simulink model "bh_proto_balance"  (R2017a)
settings: Solver=ode45  StartTime=0.0  StopTime=2  FixedStep=0.001  RelTol=1e-5  EnableMultiTasking=on
values from neighbouring files (symbols this model uses):
  L3y = res_T.L3y    [bh_pend_solve_ODE_sys.m]    (also in bh_pend_solve_ODE_sys_custom.m)
  m = res_T.mass3    [bh_pend_solve_ODE_sys_custom.m]
  N = 1 + N_steps    [bh_pend_solve_ODE_sys_custom.m]
undefined symbols (not defined in the file or in its folder): L3x, L3z, X, Y, Z
libraries: sm_lib x13, nesl_utility x8, simulink_extras x5
settings Model: Creator=bhorton  LastModifiedBy=bhorton
settings SolverCC: ZeroCrossAlgorithm=Adaptive
settings OptimizationCC: LifeSpan=inf
settings DebuggingCC: SFUnexpectedBacktrackingDiag=warning  SFNoUnconditionalDefaultTransitionDiag=warning  SFExecutionAtInitializationDiag=none
settings GRTTargetCC: TargetLangStandard=C89/C90 (ANSI)
settings ConfigComp: CovMetricSettings=dw  CovHtmlReporting=on  CovSaveCumulativeToWorkspaceVar=on  CovSaveSingleToWorkspaceVar=on  CovExternalEMLEnable=off
settings SimscapeCC: SimscapeLogDataHistory=10000  SelectedTab=Simscape Multibody
settings ExplorerConfigSet: InternalSimMechanicsExplorerSettings="<ExplorerConfiguration><canonicalview>default</canonicalview><AnimationSetting><BasePlaybackSpeed>1.0</BasePlaybackSpeed><PlaybackSpeedFactor>1.0</PlaybackSpeedFactor></AnimationSetting><TilePanel><TileInfo><Tiles Columns=\"1\" Count=\"1\" Rows=\"1\"><Column Left=\"2\" Weight=\"1\"/><Column Left=\"1585\" Weight=\"0.5\"/><Row Top=\"2\" Weight=\"1\"/><Row Top=\"911\" Weight=\"0.5005\"/><Tile Height=\"1\" Width=\"1\" X=\"0\" Y=\"0\"/></Tiles></TileInfo><SceneInfo><SceneViewer><BGColor><R>0.60000002384185791</R><G>0.60000002384185791</G><B>0.60000002384185791</B></BGColor><Camera><DoPerspective>off</DoPerspective><Position><X>0.97226610796774449</X><Y>0.24871023220719646</Y><Z>0.19848014681163439</Z></Position><Center><X>-1.1885447515069814e-08</X><Y>0.12499999495795672</Y><Z>-1.7810067587387124e-09</Z></Center><Up><X>-0.2183009159559649</X><Y>0.17550270816811642</Y><Z>0.9599705774233106</Z></Up><ViewLimDist>1</ViewLimDist><YLim>0.073618170266836078</YLim><XLim>0.12874999999999998</XLim></Camera></SceneViewer></SceneInfo></TilePanel><MechEditorPanel><Cameras/><GfxPanelCameraMap/><VideoCreator><PlaybackSpeedRatio>1.0</PlaybackSpeedRatio><FrameRate>30</FrameRate><VideoFormat>Motion JPEG AVI</VideoFormat><FrameSize>auto</FrameSize></VideoCreator></MechEditorPanel></ExplorerConfiguration>"

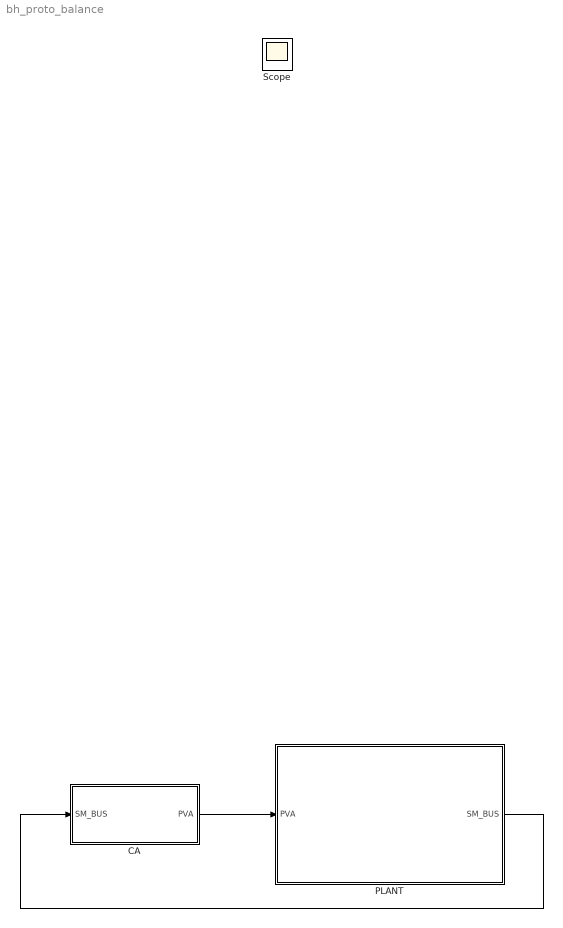
== system bh_proto_balance ==
  CA : Subsystem
  PLANT : Subsystem
  Scope : Scope
  wires:
  PLANT/1(SM_BUS) -> CA/1(SM_BUS)
  CA/1(PVA) -> PLANT/1(PVA)

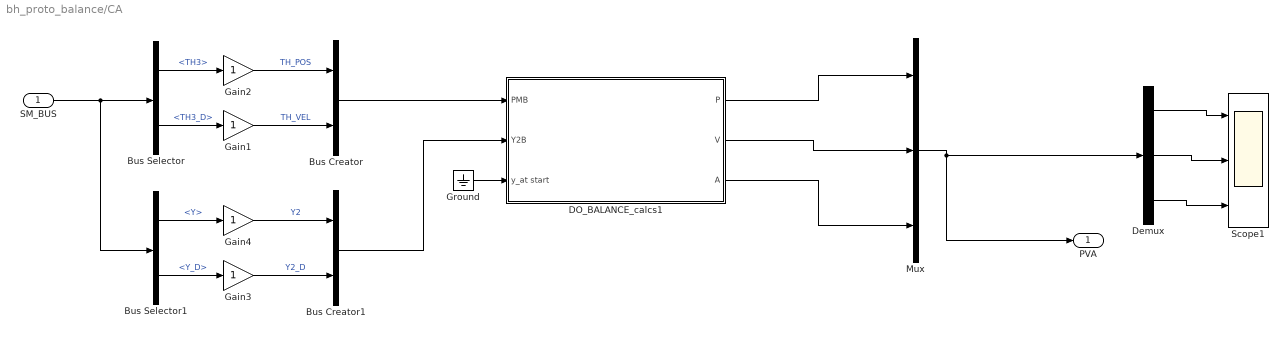
== system bh_proto_balance/CA ==
  SM_BUS : Inport
  Bus Creator : BusCreator  Inputs=2
  Bus Creator1 : BusCreator  Inputs=2
  Bus Selector : BusSelector  OutputSignals=TH3,TH3_D
  Bus Selector1 : BusSelector  OutputSignals=Y,Y_D
  DO_BALANCE_calcs1 : Subsystem  TreatAsAtomicUnit=on
  Demux : Demux  Outputs=3
  Gain{1..4} (4 alike) : Gain
  Ground : Ground
  Mux : Mux  Inputs=3
  Scope1 : Scope  NumInputPorts=3
  PVA : Outport
  wires:
  Mux/1 -> Demux/1, PVA/1
  Demux/3 -> Scope1/3
  Demux/2 -> Scope1/2
  Demux/1 -> Scope1/1
  Bus Selector/1 -> Gain2/1  "<TH3>"
  Bus Selector/2 -> Gain1/1  "<TH3_D>"
  Gain1/1 -> Bus Creator/2  "TH_VEL"
  Gain2/1 -> Bus Creator/1  "TH_POS"
  Bus Selector1/1 -> Gain4/1  "<Y>"
  Gain4/1 -> Bus Creator1/1  "Y2"
  Gain3/1 -> Bus Creator1/2  "Y2_D"
  Bus Selector1/2 -> Gain3/1  "<Y_D>"
  SM_BUS/1 -> Bus Selector1/1, Bus Selector/1
  Bus Creator/1 -> DO_BALANCE_calcs1/1(PMB)
  Bus Creator1/1 -> DO_BALANCE_calcs1/2(Y2B)
  DO_BALANCE_calcs1/1(P) -> Mux/1
  Ground/1 -> DO_BALANCE_calcs1/3(y_at start)
  DO_BALANCE_calcs1/2(V) -> Mux/2
  DO_BALANCE_calcs1/3(A) -> Mux/3

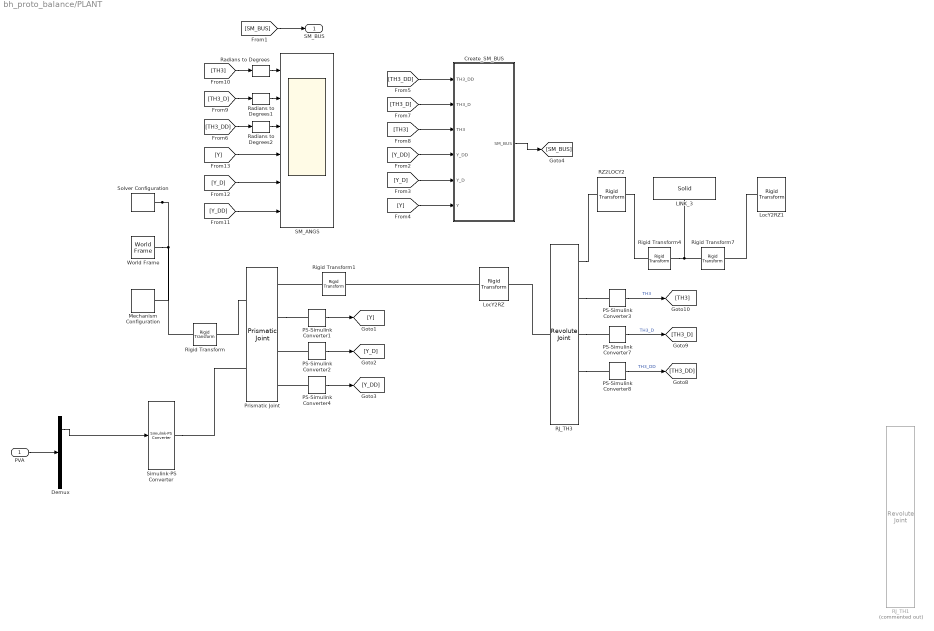
== system bh_proto_balance/PLANT ==
  PVA : Inport
  Create_SM_BUS : Subsystem
  Demux : Demux  Outputs=3
  LINK_3 : sm_lib/Body Elements/Solid  InertiaType=CalculateFromGeometry  Mass=1  MassUnits=kg  CenterOfMass=[0 0 0]  CenterOfMassUnits=m  MomentsOfInertia=[1 1 1]  MomentsOfInertiaUnits=kg*m^2  ProductsOfInertia=[0 0 0]  ProductsOfInertiaUnits=kg*m^2  DensityBased=on  Density=density  DensityUnits=kg/(m^3)  DoExposeReferenceFrame=on  SerializedFrames=<Frames/>  GraphicType=FromGeometry  MarkerShape=Sphere  MarkerSize=10  GraphicVisPropType=SimpleVisualProperties  GraphicDiffuseColor=[1.0 0.8 0.4]  GraphicSpecularColor=[0.5 0.5 0.5 1.0]  GraphicAmbientColor=[0.15 0.15 0.15 1.0]  GraphicEmissiveColor=[0.0 0.0 0.0 1.0]  GraphicShininess=75  GraphicOpacity=1.0  GeometryShape=Brick  RectangleSize=[1 1]  RectangleSizeUnits=m  BrickDimensions=[L3x, L3y, L3z ]  BrickDimensionUnits=m  CylinderRadius=1  CylinderRadiusUnits=m  CylinderLength=1  CylinderLengthUnits=m  SphereRadius=1  SphereRadiusUnits=m  EllipsoidRadii=[1 1 1]  EllipsoidRadiiUnits=m  ExtrusionCrossSection=[1 1; -1 1; -1 -1; 1 -1]  ExtrusionCrossSectionUnits=m  ExtrusionLength=1  ExtrusionLengthUnits=m  PolygonNumSides=3  PolygonOuterRadius=1  PolygonOuterRadiusUnits=m  ExtGeomFileType=STEP  ExtGeomFileUnits=m  RevolutionCrossSection=[1 1; 1 -1; 2 -1; 2 1]  RevolutionCrossSectionUnits=m  RevolutionExtent=Full  RevolutionAngle=180  RevolutionAngleUnits=deg
  LocY2RZ : sm_lib/Frames and Transforms/Rigid Transform  TranslationMethod=None  TranslationStandardOffset=0  TranslationLengthUnit=m  TranslationStandardAxis=+Z  TranslationCartesianOffset=[0 0 0]  TranslationROffset=0  TranslationROffsetUnits=m  TranslationZOffset=0  TranslationZOffsetUnits=m  TranslationThetaOffset=0  TranslationThetaOffsetUnits=deg  RotationMethod=AlignedAxes  RotationAngleUnits=deg  RotationStandardAxis=+Z  RotationAngle=0.0  RotationArbitraryAxis=[0 0 1]  FollAlignAxisA=+X  BaseAlignAxisA=+Y  FollAlignAxisB=+Y  BaseAlignAxisB=+Z  RotationSequenceAxes=FollowerAxes  RotationSequence=XYX  RotationSequenceAngles=[0 0 0]  RotationSequenceAnglesUnits=deg  RotationMatrix=[1 0 0; 0 1 0; 0 0 1]
  LocY2RZ1 : sm_lib/Frames and Transforms/Rigid Transform  TranslationMethod=None  TranslationStandardOffset=0  TranslationLengthUnit=m  TranslationStandardAxis=+Z  TranslationCartesianOffset=[0 0 0]  TranslationROffset=0  TranslationROffsetUnits=m  TranslationZOffset=0  TranslationZOffsetUnits=m  TranslationThetaOffset=0  TranslationThetaOffsetUnits=deg  RotationMethod=AlignedAxes  RotationAngleUnits=deg  RotationStandardAxis=+Z  RotationAngle=0.0  RotationArbitraryAxis=[0 0 1]  FollAlignAxisA=+X  BaseAlignAxisA=+Y  FollAlignAxisB=+Y  BaseAlignAxisB=+Z  RotationSequenceAxes=FollowerAxes  RotationSequence=XYX  RotationSequenceAngles=[0 0 0]  RotationSequenceAnglesUnits=deg  RotationMatrix=[1 0 0; 0 1 0; 0 0 1]
  Mechanism Configuration : sm_lib/Utilities/Mechanism Configuration  UniformGravity=Constant  GravityVector=[0 0 -9.80665 ]  GravityUnits=m/s^2  LinearizationDelta=1e-4
  PS-Simulink Converter1 : nesl_utility/PS-Simulink Converter  PhysicalDomain=network_engine_domain  SubClassName=ps_output  LeftPortType=input  RightPortType=output  PseudoPeriodic=off  Frequencies=[]  Unit=m  AffineConversion=off
  PS-Simulink Converter2 : nesl_utility/PS-Simulink Converter  PhysicalDomain=network_engine_domain  SubClassName=ps_output  LeftPortType=input  RightPortType=output  PseudoPeriodic=off  Frequencies=[]  Unit=m/s  AffineConversion=off
  PS-Simulink Converter3 : nesl_utility/PS-Simulink Converter  PhysicalDomain=network_engine_domain  SubClassName=ps_output  LeftPortType=input  RightPortType=output  PseudoPeriodic=off  Frequencies=[]  Unit=rad  AffineConversion=off
  PS-Simulink Converter4 : nesl_utility/PS-Simulink Converter  PhysicalDomain=network_engine_domain  SubClassName=ps_output  LeftPortType=input  RightPortType=output  PseudoPeriodic=off  Frequencies=[]  Unit=m/s^2  AffineConversion=off
  PS-Simulink Converter7 : nesl_utility/PS-Simulink Converter  PhysicalDomain=network_engine_domain  SubClassName=ps_output  LeftPortType=input  RightPortType=output  PseudoPeriodic=off  Frequencies=[]  Unit=rad/s  AffineConversion=off
  PS-Simulink Converter8 : nesl_utility/PS-Simulink Converter  PhysicalDomain=network_engine_domain  SubClassName=ps_output  LeftPortType=input  RightPortType=output  PseudoPeriodic=off  Frequencies=[]  Unit=rad/s^2  AffineConversion=off
  Prismatic Joint : sm_lib/Joints/Prismatic Joint  SenseConstraintForce=off  SenseConstraintForceX=off  SenseConstraintForceY=off  SenseConstraintForceZ=off  SenseConstraintTorque=off  SenseConstraintTorqueX=off  SenseConstraintTorqueY=off  SenseConstraintTorqueZ=off  SenseTotalForce=off  SenseTotalForceX=off  SenseTotalForceY=off  SenseTotalForceZ=off  SenseTotalTorque=off  SenseTotalTorqueX=off  SenseTotalTorqueY=off  SenseTotalTorqueZ=off  CompositeWrenchDir=FollowerOnBase  CompositeWrenchFrame=BaseFrame  EquilibriumPosition=0  EquilibriumPositionUnits=m  SpringStiffness=0  SpringStiffnessUnits=N/m  DampingCoefficient=0  DampingCoefficientUnits=N/(m/s)  TorqueActuationMode=ComputedTorque  MotionActuationMode=InputMotion  SensePosition=on  SenseVelocity=on  SenseAcceleration=on  SenseTorqueForce=off  PositionTargetSpecify=on  PositionTargetPriority=High  PositionTargetValue=0  PositionTargetValueUnits=m  VelocityTargetSpecify=on  VelocityTargetPriority=High  VelocityTargetValue=0  VelocityTargetValueUnits=m/s
  RJ_TH1 : sm_lib/Joints/Revolute Joint  Commented=on  SenseConstraintForce=on  SenseConstraintForceX=off  SenseConstraintForceY=off  SenseConstraintForceZ=off  SenseConstraintTorque=off  SenseConstraintTorqueX=off  SenseConstraintTorqueY=off  SenseConstraintTorqueZ=off  SenseTotalForce=off  SenseTotalForceX=off  SenseTotalForceY=off  SenseTotalForceZ=off  SenseTotalTorque=off  SenseTotalTorqueX=off  SenseTotalTorqueY=off  SenseTotalTorqueZ=off  CompositeWrenchDir=BaseOnFollower  CompositeWrenchFrame=BaseFrame  EquilibriumPosition=0  EquilibriumPositionUnits=deg  SpringStiffness=0  SpringStiffnessUnits=N*m/deg  DampingCoefficient=b3_damp  DampingCoefficientUnits=N*m/(rad/s)  TorqueActuationMode=NoTorque  MotionActuationMode=ComputedMotion  SensePosition=on  SenseVelocity=on  SenseAcceleration=on  SenseTorqueForce=off  PositionTargetSpecify=on  PositionTargetPriority=Low  PositionTargetValue=80  PositionTargetValueUnits=deg  VelocityTargetSpecify=on  VelocityTargetPriority=High  VelocityTargetValue=-100  VelocityTargetValueUnits=deg/s
      settings: AttributesFormatString=|
      | %<DampingCoefficient>
      | %<PositionTargetValue>
      | %<VelocityTargetValue>
  RJ_TH3 : sm_lib/Joints/Revolute Joint  SenseConstraintForce=on  SenseConstraintForceX=off  SenseConstraintForceY=off  SenseConstraintForceZ=off  SenseConstraintTorque=off  SenseConstraintTorqueX=off  SenseConstraintTorqueY=off  SenseConstraintTorqueZ=off  SenseTotalForce=off  SenseTotalForceX=off  SenseTotalForceY=off  SenseTotalForceZ=off  SenseTotalTorque=off  SenseTotalTorqueX=off  SenseTotalTorqueY=off  SenseTotalTorqueZ=off  CompositeWrenchDir=BaseOnFollower  CompositeWrenchFrame=BaseFrame  EquilibriumPosition=0  EquilibriumPositionUnits=deg  SpringStiffness=0  SpringStiffnessUnits=N*m/deg  DampingCoefficient=b3_damp  DampingCoefficientUnits=N*m/(rad/s)  TorqueActuationMode=NoTorque  MotionActuationMode=ComputedMotion  SensePosition=on  SenseVelocity=on  SenseAcceleration=on  SenseTorqueForce=off  PositionTargetSpecify=on  PositionTargetPriority=Low  PositionTargetValue=80  PositionTargetValueUnits=deg  VelocityTargetSpecify=on  VelocityTargetPriority=High  VelocityTargetValue=-350  VelocityTargetValueUnits=deg/s
      settings: AttributesFormatString=|
      | %<DampingCoefficient>
      | %<PositionTargetValue>
      | %<VelocityTargetValue>
  RZ2LOCY2 : sm_lib/Frames and Transforms/Rigid Transform  TranslationMethod=None  TranslationStandardOffset=0  TranslationLengthUnit=m  TranslationStandardAxis=+Z  TranslationCartesianOffset=[0 0 0]  TranslationROffset=0  TranslationROffsetUnits=m  TranslationZOffset=0  TranslationZOffsetUnits=m  TranslationThetaOffset=0  TranslationThetaOffsetUnits=deg  RotationMethod=AlignedAxes  RotationAngleUnits=deg  RotationStandardAxis=+Z  RotationAngle=0.0  RotationArbitraryAxis=[0 0 1]  FollAlignAxisA=+Y  BaseAlignAxisA=+X  FollAlignAxisB=+X  BaseAlignAxisB=+Z  RotationSequenceAxes=FollowerAxes  RotationSequence=XYX  RotationSequenceAngles=[0 0 0]  RotationSequenceAnglesUnits=deg  RotationMatrix=[1 0 0; 0 1 0; 0 0 1]
  Radians to Degrees : simulink_extras/Transformations/Radians to Degrees
  Radians to Degrees1 : simulink_extras/Transformations/Radians to Degrees
  Radians to Degrees2 : simulink_extras/Transformations/Radians to Degrees
  Rigid Transform : sm_lib/Frames and Transforms/Rigid Transform  TranslationMethod=None  TranslationStandardOffset=0  TranslationLengthUnit=m  TranslationStandardAxis=+Z  TranslationCartesianOffset=[0 0 0]  TranslationROffset=0  TranslationROffsetUnits=m  TranslationZOffset=0  TranslationZOffsetUnits=m  TranslationThetaOffset=0  TranslationThetaOffsetUnits=deg  RotationMethod=AlignedAxes  RotationAngleUnits=deg  RotationStandardAxis=+Z  RotationAngle=0.0  RotationArbitraryAxis=[0 0 1]  FollAlignAxisA=+X  BaseAlignAxisA=+X  FollAlignAxisB=+Z  BaseAlignAxisB=+Y  RotationSequenceAxes=FollowerAxes  RotationSequence=XYX  RotationSequenceAngles=[0 0 0]  RotationSequenceAnglesUnits=deg  RotationMatrix=[1 0 0; 0 1 0; 0 0 1]
  Rigid Transform1 : sm_lib/Frames and Transforms/Rigid Transform  TranslationMethod=None  TranslationStandardOffset=0  TranslationLengthUnit=m  TranslationStandardAxis=+Z  TranslationCartesianOffset=[0 0 0]  TranslationROffset=0  TranslationROffsetUnits=m  TranslationZOffset=0  TranslationZOffsetUnits=m  TranslationThetaOffset=0  TranslationThetaOffsetUnits=deg  RotationMethod=AlignedAxes  RotationAngleUnits=deg  RotationStandardAxis=+Z  RotationAngle=0.0  RotationArbitraryAxis=[0 0 1]  FollAlignAxisA=+X  BaseAlignAxisA=+X  FollAlignAxisB=+Y  BaseAlignAxisB=+Z  RotationSequenceAxes=FollowerAxes  RotationSequence=XYX  RotationSequenceAngles=[0 0 0]  RotationSequenceAnglesUnits=deg  RotationMatrix=[1 0 0; 0 1 0; 0 0 1]
  Rigid Transform4 : sm_lib/Frames and Transforms/Rigid Transform  TranslationMethod=StandardAxis  TranslationStandardOffset=L3y/2  TranslationLengthUnit=m  TranslationStandardAxis=+Y  TranslationCartesianOffset=[0 0 0]  TranslationROffset=0  TranslationROffsetUnits=m  TranslationZOffset=0  TranslationZOffsetUnits=m  TranslationThetaOffset=0  TranslationThetaOffsetUnits=deg  RotationMethod=None  RotationAngleUnits=deg  RotationStandardAxis=+Z  RotationAngle=0.0  RotationArbitraryAxis=[0 0 1]  FollAlignAxisA=+X  BaseAlignAxisA=+Y  FollAlignAxisB=+Y  BaseAlignAxisB=+Z  RotationSequenceAxes=FollowerAxes  RotationSequence=XYX  RotationSequenceAngles=[0 0 0]  RotationSequenceAnglesUnits=deg  RotationMatrix=[1 0 0; 0 1 0; 0 0 1]
  Rigid Transform7 : sm_lib/Frames and Transforms/Rigid Transform  TranslationMethod=StandardAxis  TranslationStandardOffset=L3y/2  TranslationLengthUnit=m  TranslationStandardAxis=+Y  TranslationCartesianOffset=[0 0 0]  TranslationROffset=0  TranslationROffsetUnits=m  TranslationZOffset=0  TranslationZOffsetUnits=m  TranslationThetaOffset=0  TranslationThetaOffsetUnits=deg  RotationMethod=None  RotationAngleUnits=deg  RotationStandardAxis=+Z  RotationAngle=0.0  RotationArbitraryAxis=[0 0 1]  FollAlignAxisA=+X  BaseAlignAxisA=+Y  FollAlignAxisB=+Y  BaseAlignAxisB=+Z  RotationSequenceAxes=FollowerAxes  RotationSequence=XYX  RotationSequenceAngles=[0 0 0]  RotationSequenceAnglesUnits=deg  RotationMatrix=[1 0 0; 0 1 0; 0 0 1]
  SM_ANGS : Scope  NumInputPorts=6
  Simulink-PS Converter : nesl_utility/Simulink-PS Converter  PhysicalDomain=network_engine_domain  SubClassName=ps_input  LeftPortType=input  RightPortType=output  PseudoPeriodic=off  Frequencies=[]  NoiseDistribution=none  NoiseParameters=[]  Unit=m  AffineConversion=off  FilteringAndDerivatives=filter  SimscapeFilterOrder=2  InputFilterTimeConstant=0.001  UdotUserProvided=2
  Solver Configuration : nesl_utility/Solver Configuration  PhysicalDomain=network_engine_domain  SubClassName=solver  LeftPortType=input  RightPortType=generic  Accelerate=off  Tones=[]  Harmonics=[]  SimulateNoise=off  Profile=off  UseLocalSampling=off  EnableSwitchedLinearOptims=on  FrequencyDomain=off  UseCCode=off  RelTol=0.001  AbsTol=1e-06  MinStep=1e-09  ToWorkspace=off  RevertToSquareIcSolve=off  NumHomotopyIterations=100  PhasorMode=off  PhasorModeNumHarmonics=1  OverrideAbsTol=off  DoDC=off  ResidualTolerance=1e-09  UseLocalSolver=off  LocalSolverChoice=NE_TRAPEZOIDAL_ADVANCER  LocalSolverSampleTime=0.01  DoFixedCost=off  MaxNonlinIter=3  MaxModeIter=2  LinearAlgebra=Sparse  DelaysMemoryBudget=1024  AutomaticFiltering=off  FilteringTimeConstant=0.001
  World Frame : sm_lib/Frames and Transforms/World Frame
  SM_BUS : Outport
  wires:
  [TH3] -> Create_SM_BUS/3(TH3)
  [Y] -> Create_SM_BUS/6(Y)
  PS-Simulink Converter7/1 -> [TH3_D]  "TH3_D"
  Demux/1 -> Simulink-PS Converter/1
  [TH3_D] -> Radians to Degrees1/1
  Create_SM_BUS/1(SM_BUS) -> [SM_BUS]
  [TH3_D] -> Create_SM_BUS/2(TH3_D)
  [TH3_DD] -> Create_SM_BUS/1(TH3_DD)
  PS-Simulink Converter3/1 -> [TH3]  "TH3"
  PS-Simulink Converter1/1 -> [Y]
  [SM_BUS] -> SM_BUS/1
  PVA/1 -> Demux/1
  [TH3] -> Radians to Degrees/1
  PS-Simulink Converter8/1 -> [TH3_DD]  "TH3_DD"
  PS-Simulink Converter4/1 -> [Y_DD]
  [Y_DD] -> Create_SM_BUS/4(Y_DD)
  PS-Simulink Converter2/1 -> [Y_D]
  [TH3_DD] -> Radians to Degrees2/1
  [Y_D] -> Create_SM_BUS/5(Y_D)
  Radians to Degrees/1 -> SM_ANGS/1
  Radians to Degrees1/1 -> SM_ANGS/2
  Radians to Degrees2/1 -> SM_ANGS/3
  [Y] -> SM_ANGS/4
  [Y_D] -> SM_ANGS/5
  [Y_DD] -> SM_ANGS/6
  connections:
  Solver Configuration/RConn1 -- World Frame/RConn1 -- Rigid Transform/LConn1 -- Mechanism Configuration/RConn1
  RZ2LOCY2/RConn1 -- Rigid Transform4/LConn1
  RJ_TH3/RConn2 -- PS-Simulink Converter3/LConn1
  Prismatic Joint/LConn1 -- Rigid Transform/RConn1
  PS-Simulink Converter4/LConn1 -- Prismatic Joint/RConn4
  LocY2RZ1/LConn1 -- Rigid Transform7/RConn1
  Prismatic Joint/RConn2 -- PS-Simulink Converter1/LConn1
  LocY2RZ/LConn1 -- Rigid Transform1/RConn1
  RJ_TH3/LConn1 -- LocY2RZ/RConn1
  Simulink-PS Converter/RConn1 -- Prismatic Joint/LConn2
  Rigid Transform4/RConn1 -- LINK_3/RConn1 -- Rigid Transform7/LConn1
  RJ_TH3/RConn3 -- PS-Simulink Converter7/LConn1
  Rigid Transform1/LConn1 -- Prismatic Joint/RConn1
  RJ_TH3/RConn4 -- PS-Simulink Converter8/LConn1
  PS-Simulink Converter2/LConn1 -- Prismatic Joint/RConn3
  RJ_TH3/RConn1 -- RZ2LOCY2/LConn1

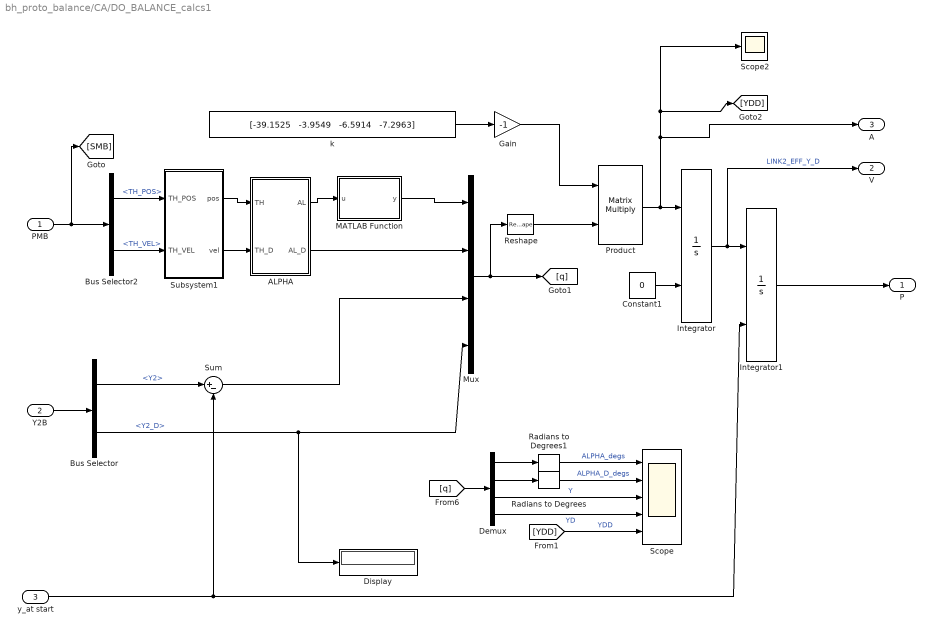
== system bh_proto_balance/CA/DO_BALANCE_calcs1 ==
  PMB : Inport
  Y2B : Inport  Port=2
  y_at start : Inport  Port=3
  ALPHA : Subsystem
  Bus Selector : BusSelector  OutputSignals=Y2,Y2_D
  Bus Selector2 : BusSelector  OutputSignals=TH_POS,TH_VEL
  Constant1 : Constant  Value=0
  Demux : Demux
  Display : Display
  Gain : Gain  Gain=-1
  Integrator : Integrator  InitialConditionSource=external
  Integrator1 : Integrator  InitialConditionSource=external
  MATLAB Function : MATLAB Function  TreatAsAtomicUnit=on
  Mux : Mux
  Product : Product  Multiplication=Matrix(*)
  Radians to Degrees : simulink_extras/Transformations/Radians to Degrees
  Radians to Degrees1 : simulink_extras/Transformations/Radians to Degrees
  Reshape : Reshape  OutputDimensionality=Column vector (2-D)
  Scope : Scope  NumInputPorts=5
  Scope2 : Scope
  Subsystem1 : Subsystem
  Sum : Sum  Inputs=|+-
  k : Constant  Value="[-39.1525   -3.9549   -6.5914   -7.2963]"  VectorParams1D=off
  P : Outport
  V : Outport  Port=2
  A : Outport  Port=3
  wires:
  Subsystem1/1(pos) -> ALPHA/1(TH)
  ALPHA/2(AL_D) -> Mux/2
  Bus Selector2/2 -> Subsystem1/2(TH_VEL)  "<TH_VEL>"
  PMB/1 -> [SMB], Bus Selector2/1
  Bus Selector2/1 -> Subsystem1/1(TH_POS)  "<TH_POS>"
  Mux/1 -> Reshape/1, [q]
  k/1 -> Gain/1
  Reshape/1 -> Product/2
  Gain/1 -> Product/1
  Product/1 -> A/1, [YDD], Scope2/1, Integrator/1
  Constant1/1 -> Integrator/2
  y_at start/1 -> Sum/2, Integrator1/2
  Radians to Degrees1/1 -> Scope/1  "ALPHA_degs"
  Radians to Degrees/1 -> Scope/2  "ALPHA_D_degs"
  MATLAB Function/1(y) -> Mux/1
  ALPHA/1(AL) -> MATLAB Function/1(u)
  Subsystem1/2(vel) -> ALPHA/2(TH_D)
  Y2B/1 -> Bus Selector/1
  Bus Selector/2 -> Display/1, Mux/4  "<Y2_D>"
  Bus Selector/1 -> Sum/1  "<Y2>"
  Integrator/1 -> V/1, Integrator1/1  "LINK2_EFF_Y_D"
  Demux/4 -> Scope/4  "YD"
  Demux/3 -> Scope/3  "Y"
  Demux/2 -> Radians to Degrees/1
  Demux/1 -> Radians to Degrees1/1
  [q] -> Demux/1
  Sum/1 -> Mux/3
  Integrator1/1 -> P/1
  [YDD] -> Scope/5  "YDD"

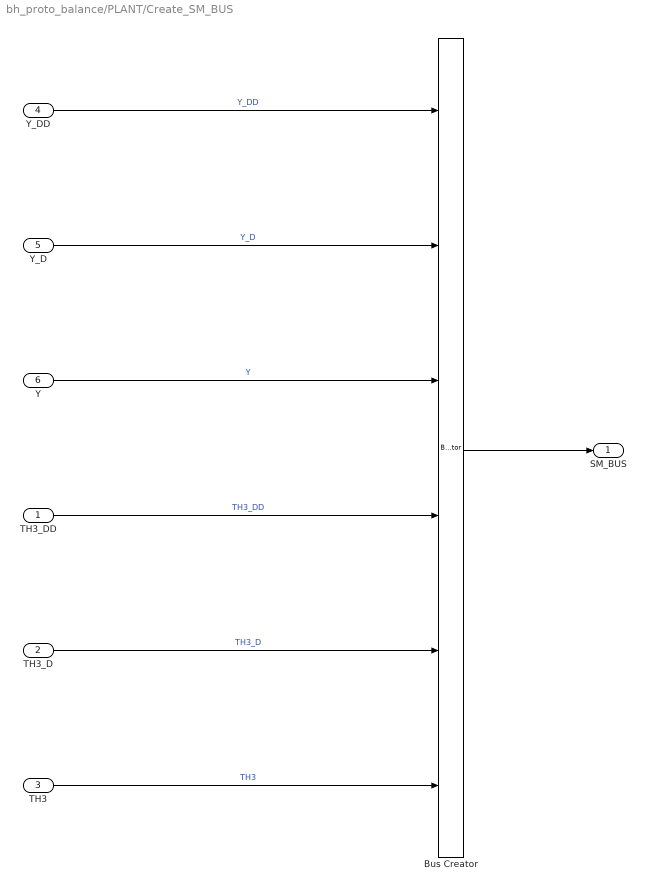
== system bh_proto_balance/PLANT/Create_SM_BUS ==
  TH3_DD : Inport
  TH3_D : Inport  Port=2
  TH3 : Inport  Port=3
  Y_DD : Inport  Port=4
  Y_D : Inport  Port=5
  Y : Inport  Port=6
  Bus Creator : BusCreator  Inputs=6
  SM_BUS : Outport
  wires:
  Bus Creator/1 -> SM_BUS/1
  TH3/1 -> Bus Creator/6  "TH3"
  TH3_D/1 -> Bus Creator/5  "TH3_D"
  TH3_DD/1 -> Bus Creator/4  "TH3_DD"
  Y_D/1 -> Bus Creator/2  "Y_D"
  Y/1 -> Bus Creator/3  "Y"
  Y_DD/1 -> Bus Creator/1  "Y_DD"

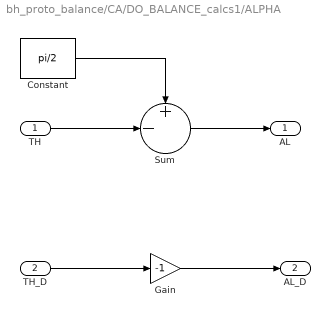
== system bh_proto_balance/CA/DO_BALANCE_calcs1/ALPHA ==
  TH : Inport
  TH_D : Inport  Port=2
  Constant : Constant  Value=pi/2
  Gain : Gain  Gain=-1
  Sum : Sum  Inputs=+-|
  AL : Outport
  AL_D : Outport  Port=2
  wires:
  TH/1 -> Sum/2
  Constant/1 -> Sum/1
  Sum/1 -> AL/1
  TH_D/1 -> Gain/1
  Gain/1 -> AL_D/1

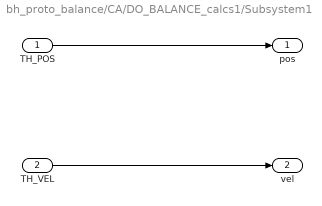
== system bh_proto_balance/CA/DO_BALANCE_calcs1/Subsystem1 ==
  TH_POS : Inport
  TH_VEL : Inport  Port=2
  pos : Outport
  vel : Outport  Port=2
  wires:
  TH_POS/1 -> pos/1
  TH_VEL/1 -> vel/1

== matlab function bh_proto_balance/CA/DO_BALANCE_calcs1/MATLAB Function ==
  data: u input; y output
function y = fcn(u)
coder.extrinsic('wrapToPi');
y = 0;
y = wrapToPi(u);
